simulink library "Bibliothek_FHDO_V1"  (R2025b)
settings: Solver=VariableStepAuto  StartTime=0.0  StopTime=10.0  RelTol=1e-3
libraries: $bdroot x5
settings Model: Creator=goessling  LastModifiedBy=henni

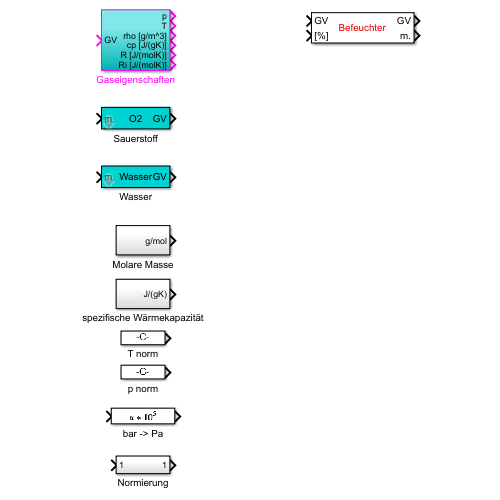
[thumbnail: Simulink's stored preview of the top-level diagram]
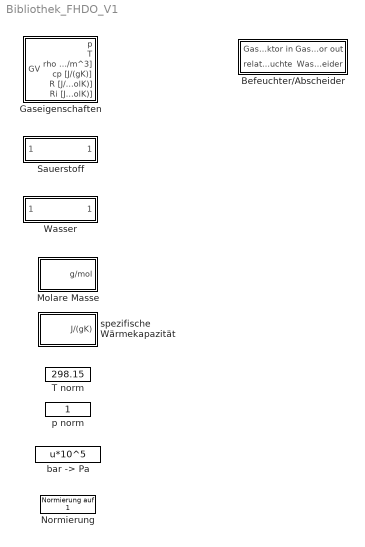
== system Bibliothek_FHDO_V1 ==
  Befeuchter/Abscheider : Subsystem
      mask Display:
      | color('red')
      | disp('Befeuchter');
      | 
      | color('black')
      | port_label('output', 1, 'GV')
      | port_label('output', 2, 'm.')
      | port_label('input', 1, 'GV')
      | port_label('input', 2, '[%]')
  Gaseigenschaften : Subsystem
  Molare Masse : Subsystem
  Normierung : $bdroot/Sauerstoff/Normierung auf 1  SystemSampleTime=-1  VariantActivationTime=update diagram  EmptyChoice=off  PassThrough=off  PassThroughVariantControl=(default)  EmptyChoiceVariantControl=(default)  AllowFlexibleInterface=on  Latency=0  AutoFrameSizeCalculation=off
  Sauerstoff : Subsystem  mask{p=1, T=25}
      mask prompts: p "p [bar]"; T "T [°C]"
      mask Display:
      | disp('O2')
      | 
      | port_label ('input', 1, 'm.')
      | port_label ('output', 1, 'GV')
  T norm : Constant  Value=298.15
  Wasser : Subsystem  mask{p=1, T=25}
      mask prompts: p "p [bar]"; T "T [°C]"
      mask Display:
      | disp('Wasser')
      | 
      | port_label ('input', 1, 'm.')
      | port_label ('output', 1, 'GV')
  "bar -> Pa" : Fcn  Expr=u*10^5
  p norm : Constant
  spezifische Wärmekapazität : Subsystem

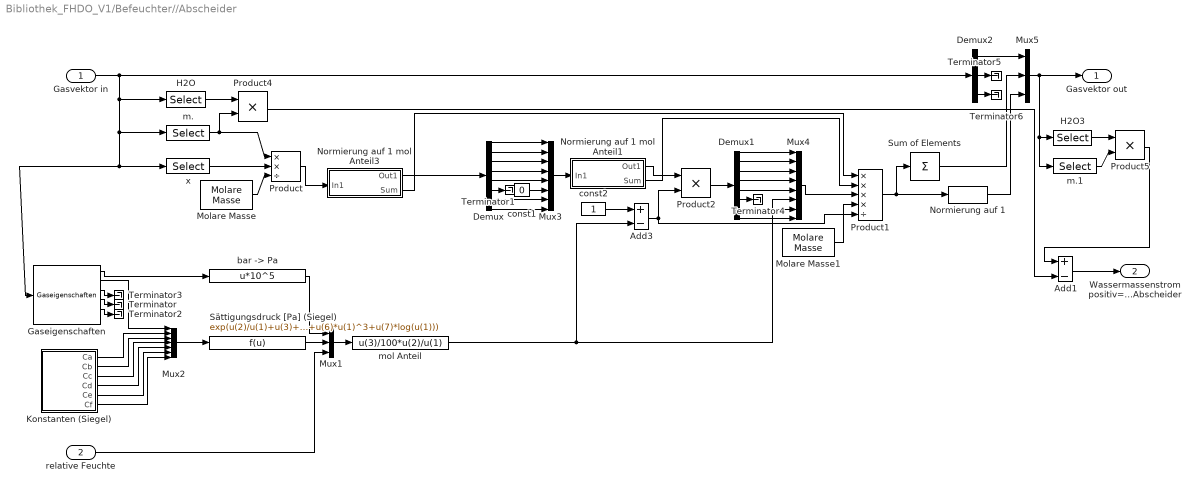
== system Bibliothek_FHDO_V1/Befeuchter//Abscheider ==
  Gasvektor in : Inport
  relative Feuchte : Inport  Port=2
  Add1 : Sum  Inputs=+-
  Add3 : Sum  Inputs=+-
  Demux : Demux  Outputs=8
  Demux1 : Demux  Outputs=8
  Demux2 : Demux  Outputs=[2 1 8]
  Gaseigenschaften : $bdroot/Gaseigenschaften  SystemSampleTime=-1  VariantActivationTime=update diagram  AllowFlexibleInterface=on  Latency=0  AutoFrameSizeCalculation=off
  H2O : Selector  InputPortWidth=11  IndexOptions=Index vector (dialog)  Indices=9  OutputSizes=1
  H2O3 : Selector  InputPortWidth=11  IndexOptions=Index vector (dialog)  Indices=9  OutputSizes=1
  Konstanten (Siegel) : Subsystem
  Molare Masse : $bdroot/Molare Masse  SystemSampleTime=-1  VariantActivationTime=update diagram  AllowFlexibleInterface=on  Latency=0  AutoFrameSizeCalculation=off
  Molare Masse1 : $bdroot/Molare Masse  SystemSampleTime=-1  VariantActivationTime=update diagram  AllowFlexibleInterface=on  Latency=0  AutoFrameSizeCalculation=off
  Mux1 : Mux  Inputs=3
  Mux2 : Mux  Inputs=7
  Mux3 : Mux  Inputs=8
  Mux4 : Mux  Inputs=8
  Mux5 : Mux  Inputs=3
  Normierung auf 1 : $bdroot/Sauerstoff/Normierung auf 1  SystemSampleTime=-1  VariantActivationTime=update diagram  AllowFlexibleInterface=on  Latency=0  AutoFrameSizeCalculation=off
  Normierung auf 1 mol Anteil1 : Subsystem
  Normierung auf 1 mol Anteil3 : Subsystem
  Product : Product  Inputs=**/  RndMeth=Zero
  Product1 : Product  Inputs=****/  RndMeth=Zero
  Product2 : Product  RndMeth=Zero
  Product4 : Product  RndMeth=Zero
  Product5 : Product  RndMeth=Zero
  Sum of Elements : Sum  Inputs=+
  Sättigungsdruck [Pa] (Siegel) : Fcn  Expr=exp(u(2)/u(1)+u(3)+u(4)*u(1)+u(5)*u(1)^2+u(6)*u(1)^3+u(7)*log(u(1)))
  Terminator{,1..6} (7 alike) : Terminator
  "bar -> Pa" : Fcn  Expr=u*10^5
  const1 : Constant  Value=0
  const2 : Constant
  m. : Selector  InputPortWidth=11  IndexOptions=Index vector (dialog)  Indices=3  OutputSizes=1
  m.1 : Selector  InputPortWidth=11  IndexOptions=Index vector (dialog)  Indices=3  OutputSizes=1
  mol Anteil : Fcn  Expr=u(3)/100*u(2)/u(1)
  x : Selector  InputPortWidth=11  IndexOptions=Index vector (dialog)  Indices=[4 5 6 7 8 9 10 11]  OutputSizes=1
  Gasvektor out : Outport
  Wassermassenstrom positiv=Befeuchter negativ=Abscheider : Outport  Port=2
  wires:
  Demux1/8 -> Mux4/8
  Demux1/7 -> Mux4/7
  Demux1/5 -> Mux4/5
  Demux1/4 -> Mux4/4
  Demux1/3 -> Mux4/3
  Demux1/2 -> Mux4/2
  Demux1/1 -> Mux4/1
  Demux1/6 -> Terminator4/1
  Demux/8 -> Mux3/8
  Demux/7 -> Mux3/7
  Demux/5 -> Mux3/5
  Demux/4 -> Mux3/4
  Demux/3 -> Mux3/3
  Demux/2 -> Mux3/2
  Demux/1 -> Mux3/1
  const1/1 -> Mux3/6
  Demux/6 -> Terminator1/1
  Add1/1 -> Wassermassenstrom positiv=Befeuchter negativ=Abscheider/1
  Product4/1 -> Add1/2
  Product5/1 -> Add1/1
  H2O3/1 -> Product5/1
  m.1/1 -> Product5/2
  H2O/1 -> Product4/1
  Normierung auf 1 mol Anteil1/2(Sum) -> Product1/2
  Normierung auf 1 mol Anteil3/2(Sum) -> Product1/1
  Normierung auf 1 mol Anteil3/1(Out1) -> Demux/1
  Normierung auf 1/1 -> Mux5/3
  Mux5/1 -> m.1/1, H2O3/1, Gasvektor out/1
  Demux2/3 -> Terminator6/1
  Demux2/2 -> Terminator5/1
  Product1/1 -> Normierung auf 1/1, Sum of Elements/1
  Sum of Elements/1 -> Mux5/2
  Demux2/1 -> Mux5/1
  m./1 -> Product/1, Product4/2
  Molare Masse1/1 -> Product1/4
  Mux4/1 -> Product1/3
  Product2/1 -> Demux1/1
  Add3/1 -> Product1/5, Product2/2
  Normierung auf 1 mol Anteil1/1(Out1) -> Product2/1
  mol Anteil/1 -> Mux4/6, Add3/2
  const2/1 -> Add3/1
  Mux3/1 -> Normierung auf 1 mol Anteil1/1(In1)
  Product/1 -> Normierung auf 1 mol Anteil3/1(In1)
  Molare Masse/1 -> Product/3
  x/1 -> Product/2
  "bar -> Pa"/1 -> Mux1/1
  relative Feuchte/1 -> Mux1/3
  Mux1/1 -> mol Anteil/1
  Sättigungsdruck [Pa] (Siegel)/1 -> Mux1/2
  Mux2/1 -> Sättigungsdruck [Pa] (Siegel)/1
  Gaseigenschaften/5 -> Terminator2/1
  Gaseigenschaften/4 -> Terminator/1
  Gaseigenschaften/3 -> Terminator3/1
  Gaseigenschaften/1 -> "bar -> Pa"/1
  Konstanten (Siegel)/6(Cf) -> Mux2/7
  Konstanten (Siegel)/5(Ce) -> Mux2/6
  Konstanten (Siegel)/4(Cd) -> Mux2/5
  Konstanten (Siegel)/3(Cc) -> Mux2/4
  Konstanten (Siegel)/2(Cb) -> Mux2/3
  Konstanten (Siegel)/1(Ca) -> Mux2/2
  Gaseigenschaften/2 -> Mux2/1
  Gasvektor in/1 -> H2O/1, Gaseigenschaften/1, x/1, m./1, Demux2/1

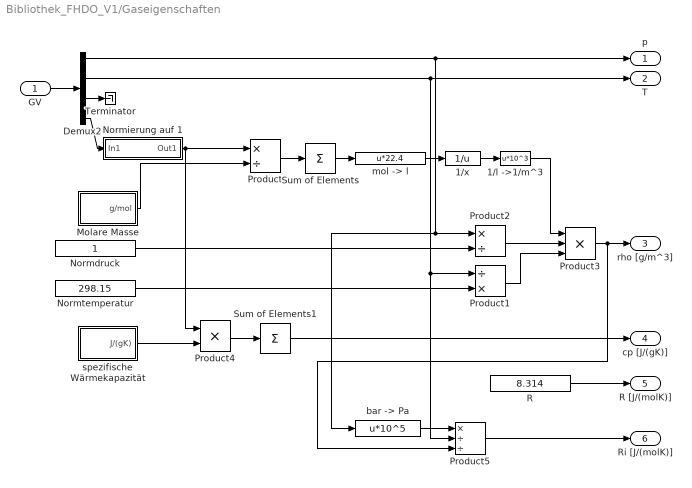
== system Bibliothek_FHDO_V1/Gaseigenschaften ==
  GV : Inport
  1/l ->1/m^3 : Fcn  Expr=u*10^3
  1/x : Fcn  Expr=1/u
  Demux2 : Demux  Outputs=[1 1 1 4]
  Molare Masse : Subsystem
  Normdruck : Constant
  Normierung auf 1 : Subsystem
  Normtemperatur : Constant  Value=298.15
  Product : Product  Inputs=*/  RndMeth=Zero
  Product1 : Product  Inputs=/*  RndMeth=Zero
  Product2 : Product  Inputs=*/  RndMeth=Zero
  Product3 : Product  Inputs=3  RndMeth=Zero
  Product4 : Product  RndMeth=Zero
  Product5 : Product  Inputs=*//
  R : Constant  Value=8.314
  Sum of Elements : Sum  Inputs=+
  Sum of Elements1 : Sum  Inputs=+
  Terminator : Terminator
  "bar -> Pa" : Fcn  Expr=u*10^5
  "mol -> l" : Fcn  Expr=u*22.4
  spezifische Wärmekapazität : Subsystem
  p : Outport
  T : Outport  Port=2
  rho [g/m^3] : Outport  Port=3
  cp [J/(gK)] : Outport  Port=4
  R [J/(molK)] : Outport  Port=5
  Ri [J/(molK)] : Outport  Port=6
  wires:
  R/1 -> R [J/(molK)]/1
  Sum of Elements1/1 -> cp [J/(gK)]/1
  Product4/1 -> Sum of Elements1/1
  spezifische Wärmekapazität/1(J/(gK)) -> Product4/2
  Sum of Elements/1 -> "mol -> l"/1
  "mol -> l"/1 -> 1/x/1
  Demux2/3 -> Terminator/1
  Product3/1 -> Product5/3, rho [g/m^3]/1
  Product1/1 -> Product3/3
  Product2/1 -> Product3/2
  Normtemperatur/1 -> Product1/2
  Normdruck/1 -> Product2/2
  Product/1 -> Sum of Elements/1
  Normierung auf 1/1(Out1) -> Product4/1, Product/1
  Molare Masse/1(g/mol) -> Product/2
  Demux2/4 -> Normierung auf 1/1(In1)
  Demux2/2 -> Product5/2, Product1/1, T/1
  Demux2/1 -> Product2/1, "bar -> Pa"/1, p/1
  GV/1 -> Demux2/1
  1/x/1 -> 1/l ->1/m^3/1
  1/l ->1/m^3/1 -> Product3/1
  Product5/1 -> Ri [J/(molK)]/1
  "bar -> Pa"/1 -> Product5/1

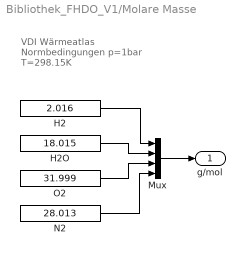
== system Bibliothek_FHDO_V1/Molare Masse ==
  note: VDI Wärmeatlas
      | Normbedingungen
      | p=1bar
      | T=298.15K
  H2 : Constant  Value=2.016
  H2O : Constant  Value=18.015
  Mux : Mux
  N2 : Constant  Value=28.013
  O2 : Constant  Value=31.999
  g/mol : Outport
  wires:
  Mux/1 -> g/mol/1
  H2O/1 -> Mux/2
  O2/1 -> Mux/3
  H2/1 -> Mux/1
  N2/1 -> Mux/4

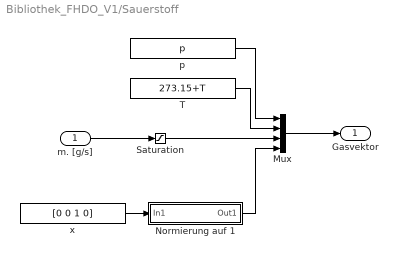
== system Bibliothek_FHDO_V1/Sauerstoff ==
  m. [g/s] : Inport
  Mux : Mux
  Normierung auf 1 : Subsystem  AncestorBlock=eigene_library_4komp/Normierung auf 1
  Saturation : Saturate  UpperLimit=inf  LowerLimit=eps
  T : Constant  Value=273.15+T
  p : Constant  Value=p
  x : Constant  Value=[0 0 1 0]
  Gasvektor : Outport
  wires:
  x/1 -> Normierung auf 1/1(In1)
  p/1 -> Mux/1
  T/1 -> Mux/2
  m. [g/s]/1 -> Saturation/1
  Normierung auf 1/1(Out1) -> Mux/4
  Mux/1 -> Gasvektor/1
  Saturation/1 -> Mux/3

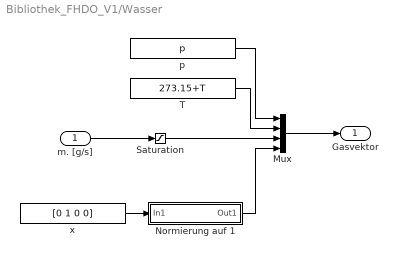
== system Bibliothek_FHDO_V1/Wasser ==
  m. [g/s] : Inport
  Mux : Mux
  Normierung auf 1 : Subsystem  AncestorBlock=eigene_library_4komp/Normierung auf 1
  Saturation : Saturate  UpperLimit=inf  LowerLimit=eps
  T : Constant  Value=273.15+T
  p : Constant  Value=p
  x : Constant  Value=[0 1 0 0]
  Gasvektor : Outport
  wires:
  x/1 -> Normierung auf 1/1(In1)
  p/1 -> Mux/1
  T/1 -> Mux/2
  m. [g/s]/1 -> Saturation/1
  Normierung auf 1/1(Out1) -> Mux/4
  Mux/1 -> Gasvektor/1
  Saturation/1 -> Mux/3

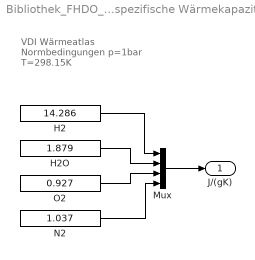
== system Bibliothek_FHDO_V1/spezifische Wärmekapazität ==
  note: VDI Wärmeatlas
      | Normbedingungen
      | p=1bar
      | T=298.15K
  H2 : Constant  Value=14.286
  H2O : Constant  Value=1.879
  Mux : Mux
  N2 : Constant  Value=1.037
  O2 : Constant  Value=0.927
  J/(gK) : Outport
  wires:
  Mux/1 -> J/(gK)/1
  H2O/1 -> Mux/2
  O2/1 -> Mux/3
  H2/1 -> Mux/1
  N2/1 -> Mux/4

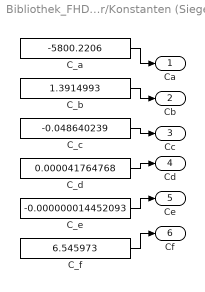
== system Bibliothek_FHDO_V1/Befeuchter//Abscheider/Konstanten (Siegel) ==
  C_a : Constant  Value=-5800.2206
  C_b : Constant  Value=1.3914993
  C_c : Constant  Value=-0.048640239
  C_d : Constant  Value=0.000041764768
  C_e : Constant  Value=-0.000000014452093
  C_f : Constant  Value=6.545973
  Ca : Outport
  Cb : Outport  Port=2
  Cc : Outport  Port=3
  Cd : Outport  Port=4
  Ce : Outport  Port=5
  Cf : Outport  Port=6
  wires:
  C_f/1 -> Cf/1
  C_e/1 -> Ce/1
  C_d/1 -> Cd/1
  C_c/1 -> Cc/1
  C_b/1 -> Cb/1
  C_a/1 -> Ca/1

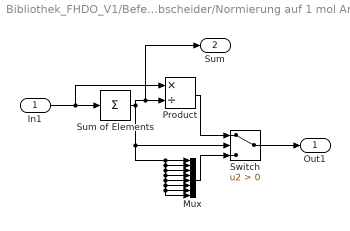
== system Bibliothek_FHDO_V1/Befeuchter//Abscheider/Normierung auf 1 mol Anteil1 ==
  In1 : Inport
  Mux : Mux  Inputs=8
  Product : Product  Inputs=*/  RndMeth=Zero
  Sum of Elements : Sum  Inputs=+
  Switch : Switch  Criteria=u2 > Threshold  SaturateOnIntegerOverflow=off  InputSameDT=off
  Out1 : Outport
  Sum : Outport  Port=2
  wires:
  In1/1 -> Sum of Elements/1, Product/1
  Sum of Elements/1 -> Switch/2, Mux/1, Mux/8, Mux/7, Mux/6, Mux/5, Mux/4, Mux/3, Mux/2, Product/2, Sum/1
  Product/1 -> Switch/1
  Switch/1 -> Out1/1
  Mux/1 -> Switch/3

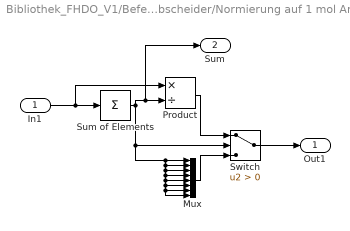
== system Bibliothek_FHDO_V1/Befeuchter//Abscheider/Normierung auf 1 mol Anteil3 ==
  In1 : Inport
  Mux : Mux  Inputs=8
  Product : Product  Inputs=*/  RndMeth=Zero
  Sum of Elements : Sum  Inputs=+
  Switch : Switch  Criteria=u2 > Threshold  SaturateOnIntegerOverflow=off  InputSameDT=off
  Out1 : Outport
  Sum : Outport  Port=2
  wires:
  Mux/1 -> Switch/3
  Switch/1 -> Out1/1
  Product/1 -> Switch/1
  Sum of Elements/1 -> Sum/1, Product/2, Mux/2, Mux/3, Mux/4, Mux/5, Mux/6, Mux/7, Mux/8, Mux/1, Switch/2
  In1/1 -> Product/1, Sum of Elements/1

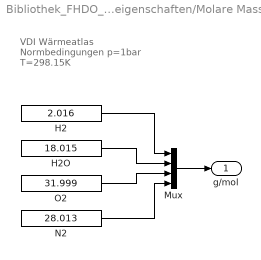
== system Bibliothek_FHDO_V1/Gaseigenschaften/Molare Masse ==
  note: VDI Wärmeatlas
      | Normbedingungen
      | p=1bar
      | T=298.15K
  H2 : Constant  Value=2.016
  H2O : Constant  Value=18.015
  Mux : Mux
  N2 : Constant  Value=28.013
  O2 : Constant  Value=31.999
  g/mol : Outport
  wires:
  Mux/1 -> g/mol/1
  H2O/1 -> Mux/2
  O2/1 -> Mux/3
  H2/1 -> Mux/1
  N2/1 -> Mux/4

== system Bibliothek_FHDO_V1/Gaseigenschaften/Normierung auf 1 ==
  In1 : Inport
  Product : Product  Inputs=*/  RndMeth=Zero
  Sum of Elements : Sum  Inputs=+
  Out1 : Outport
  wires:
  In1/1 -> Sum of Elements/1, Product/1
  Sum of Elements/1 -> Product/2
  Product/1 -> Out1/1

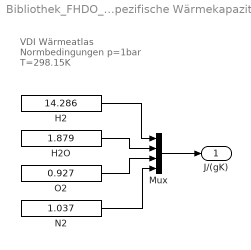
== system Bibliothek_FHDO_V1/Gaseigenschaften/spezifische Wärmekapazität ==
  note: VDI Wärmeatlas
      | Normbedingungen
      | p=1bar
      | T=298.15K
  H2 : Constant  Value=14.286
  H2O : Constant  Value=1.879
  Mux : Mux
  N2 : Constant  Value=1.037
  O2 : Constant  Value=0.927
  J/(gK) : Outport
  wires:
  Mux/1 -> J/(gK)/1
  H2O/1 -> Mux/2
  O2/1 -> Mux/3
  H2/1 -> Mux/1
  N2/1 -> Mux/4

== system Bibliothek_FHDO_V1/Sauerstoff/Normierung auf 1 ==
  In1 : Inport
  Product : Product  Inputs=*/  RndMeth=Zero
  Sum of Elements : Sum  Inputs=+
  Out1 : Outport
  wires:
  Product/1 -> Out1/1
  Sum of Elements/1 -> Product/2
  In1/1 -> Product/1, Sum of Elements/1

== system Bibliothek_FHDO_V1/Wasser/Normierung auf 1 ==
  In1 : Inport
  Product : Product  Inputs=*/  RndMeth=Zero
  Sum of Elements : Sum  Inputs=+
  Out1 : Outport
  wires:
  Product/1 -> Out1/1
  Sum of Elements/1 -> Product/2
  In1/1 -> Product/1, Sum of Elements/1
